simulink model "Simulacion_CyD"  (R2017b)
settings: Solver=VariableStepAuto  StartTime=0.0  StopTime=10.0  RelTol=1e-3
values from neighbouring files (symbols this model uses):
  dc = [.0000001 .0001 1]    [Practica2Control3.m]
  nc = 1    [Practica2Control3.m]
undefined symbols (not defined in the file or in its folder): dd, nd
settings Model: Creator=Agustin  LastModifiedBy=Agustin

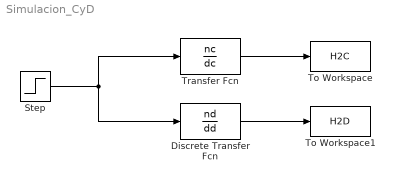
== system Simulacion_CyD ==
  Discrete Transfer Fcn : DiscreteTransferFcn  Numerator=nd  Denominator=dd  SampleTime=.5
  Step : Step  Time=0  SampleTime=0
  To Workspace : ToWorkspace  VariableName=H2C  SaveFormat=Timeseries  SampleTime=-1
  To Workspace1 : ToWorkspace  VariableName=H2D  SaveFormat=Timeseries  SampleTime=-1
  Transfer Fcn : TransferFcn  Numerator=nc  Denominator=dc
  wires:
  Transfer Fcn/1 -> To Workspace/1
  Step/1 -> Discrete Transfer Fcn/1, Transfer Fcn/1
  Discrete Transfer Fcn/1 -> To Workspace1/1
